simulink model "fuzzyPD_FINAL"  (R2020b)
settings: Solver=VariableStepAuto  StartTime=0.0  StopTime=100  RelTol=1e-3
libraries: fuzblock x1
settings Model: Creator=Daniela  LastModifiedBy=Daniela

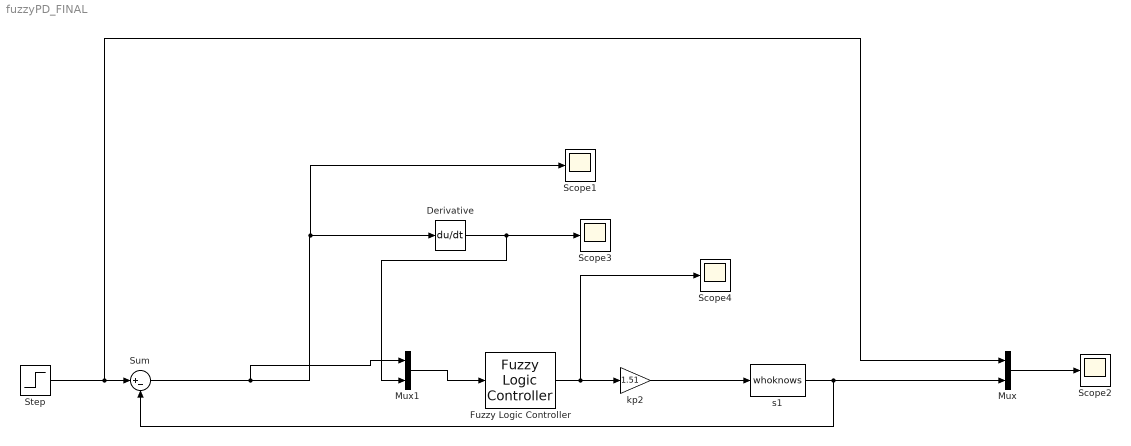
== system fuzzyPD_FINAL ==
  Derivative : Derivative
  Fuzzy Logic Controller : fuzblock/Fuzzy Logic  Controller  FIS='FuzzyPD_Final.fis'  OutputSampleNumber=101  DataType=double  FuzzifiedInputs=off  RuleFiringStrengths=off  RuleOutputs=off  AggregatedOutputs=off  SimulateUsing=Interpreted execution  OutOfRangeInputValueMessage=warning  NoRuleFiredMessage=warning  EmptyOutputFuzzySetMessage=warning
  Mux : Mux  Inputs=2
  Mux1 : Mux  Inputs=2
  Scope{1..4} (4 alike) : Scope
  Step : Step  SampleTime=0
  Sum : Sum  Inputs=|+-
  kp2 : Gain  Gain=1.51
  s1 : M-S-Function  FunctionName=whoknows  Parameters=L, P1, P2, T, R  mask{L=7, P1=0, P2=7, T=2, R=0}
      mask prompts: L "Laboratorio"; P1 "Primer digito del Puesto"; P2 "Segundo digito del Puesto"; T "Tipo de Planta"; R "Ruido"
      mask Display: disp('Sistema')
  wires:
  Mux1/1 -> Fuzzy Logic Controller/1
  Derivative/1 -> Mux1/2, Scope3/1
  Mux/1 -> Scope2/1
  Sum/1 -> Mux1/1, Scope1/1, Derivative/1
  Step/1 -> Sum/1, Mux/1
  s1/1 -> Mux/2, Sum/2
  kp2/1 -> s1/1
  Fuzzy Logic Controller/1 -> kp2/1, Scope4/1
